simulink model "navion_demo1"  (Simulink 4.0)
settings: Solver=ode4  StartTime=0.0  StopTime=120  FixedStep=0.02  RelTol=1e-3
libraries: simulink_extras x3, aerosimlib x1
settings Model: LastModifiedBy=mariusn  SaveTime=off  SaveOutput=off  LimitDataPoints=off  UnconnectedInputMsg=none  UnconnectedOutputMsg=none  UnconnectedLineMsg=none  BlockReductionOpt=off

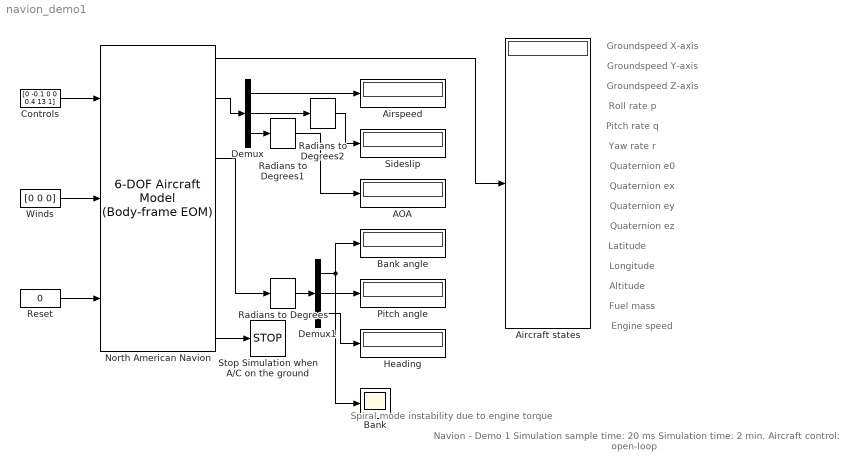
== system navion_demo1 ==
  note: Groundspeed X-axis
  note: Groundspeed Y-axis
  note: Groundspeed Z-axis
  note: Roll rate p
  note: Pitch rate q
  note: Yaw rate r
  note: Quaternion e0
  note: Quaternion ex
  note: Quaternion ey
  note: Quaternion ez
  note: Latitude
  note: Longitude
  note: Altitude
  note: Fuel mass
  note: Engine speed
  note: Navion - Demo 1
      | Simulation sample time: 20 ms
      | Simulation time: 2 min.
      | Aircraft control: open-loop
  note: Spiral mode instability
      | due to engine torque
  AOA : Display
      settings: Format=short
  Aircraft states : Display
      settings: Format=short
  Airspeed : Display
      settings: Format=short
  Bank : Scope
      settings: TimeRange=120  YMin=-100  YMax=0  SaveToWorkspace=off  SaveName=ScopeData  MaxDataPoints=5000
  Bank angle : Display
      settings: Format=short
  Controls : Constant  Value=[0 -0.1 0 0 0.4 13 1]
  Demux : Demux  Outputs=3  BusSelectionMode=off
  Demux1 : Demux  Outputs=3  BusSelectionMode=off
  Heading : Display
      settings: Format=short
  North American Navion : aerosimlib/Complete Aircraft/6-DOF Aircraft Model (Body-frame EOM)  aircraftcfg='navioncfg.mat'  VelocitiesIni=[50 0 0]'  RatesIni=[0 0 0]'  QuaternionsIni=[1 0 0 0]'  PositionIni=[45*pi/180 -122*pi/180 1000]'  FuelIni=200  OmegaIni=2400*pi/30  GndAlt=20  wmmfile='C:\Program Files\AeroSim\wmm.cof'  dmy=[09 01 2002]  tsamp=0.02
  Pitch angle : Display
      settings: Format=short
  Radians to Degrees : simulink_extras/Transformations/Radians to Degrees
  Radians to Degrees1 : simulink_extras/Transformations/Radians to Degrees
  Radians to Degrees2 : simulink_extras/Transformations/Radians to Degrees
  Reset : Constant  Value=0
  Sideslip : Display
      settings: Format=short
  Stop Simulation when A/C on the ground : Stop
  Winds : Constant  Value=[0 0 0]
  wires:
  Controls/1 -> North American Navion/1
  Winds/1 -> North American Navion/2
  Reset/1 -> North American Navion/3
  North American Navion/1 -> Aircraft states/1
  North American Navion/6 -> Radians to Degrees/1
  North American Navion/3 -> Demux/1
  Demux/3 -> Radians to Degrees1/1
  Demux/2 -> Radians to Degrees2/1
  Demux/1 -> Airspeed/1
  Radians to Degrees2/1 -> Sideslip/1
  Radians to Degrees1/1 -> AOA/1
  North American Navion/15 -> Stop Simulation when A/C on the ground/1
  Radians to Degrees/1 -> Demux1/1
  Demux1/2 -> Pitch angle/1
  Demux1/3 -> Heading/1
  Demux1/1 -> Bank/1, Bank angle/1
